simulink model "hydraulic_motor"  (R2013b)
settings: Solver=ode45  StartTime=0.0  StopTime=t_end  MaxStep=0.001  RelTol=1e-3
values from neighbouring files (symbols this model uses):
  b = 1e-3    (= 0.001)    [Hydraulic_script.m]
  C = 1e-12    [Hydraulic_script.m]
  I = 20000    [Hydraulic_script.m]
  J = r^2*100/(i^2)    (= 0.00907029478458)    [Hydraulic_script.m]
  P = 55000    [Hydraulic_script.m]
  target_angular_velocity = 210    [Hydraulic_script.m]
  Vr = 8.2e-6    (= 8.2e-06)    [Hydraulic_script.m]
settings Model: Creator=tlantela  LastModifiedBy=Tapio
settings OptimizationCC: SimCompilerOptimization=off
settings DebuggingCC: UnderspecifiedInitializationDetection=Simplified  MergeDetectMultiDrivingBlocksExec=error  FrameProcessingCompatibilityMsg=error
settings RTWCC: RTWCompilerOptimization=off
settings GRTTargetCC: TargetLangStandard=C89/C90 (ANSI)  CodeReplacementLibrary=None  CPPClassGenCompliant=on

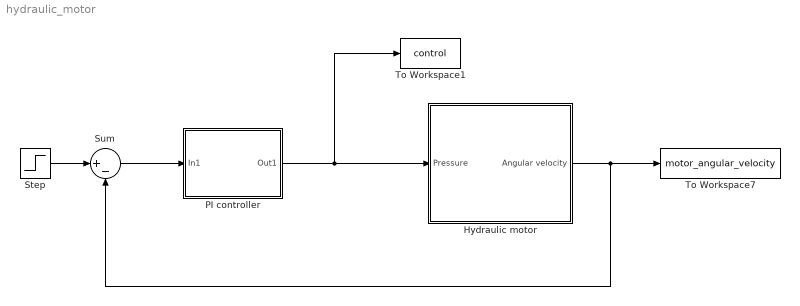
== system hydraulic_motor ==
  Hydraulic motor : Subsystem
  PI controller : Subsystem
  Step : Step  Time=0  After=target_angular_velocity  SampleTime=0
  Sum : Sum  Inputs=|+-
  To Workspace1 : ToWorkspace  VariableName=control  SampleTime=-1  SaveFormat=Timeseries
  To Workspace7 : ToWorkspace  VariableName=motor_angular_velocity  SampleTime=-1  SaveFormat=Timeseries
  wires:
  Hydraulic motor/1(Angular velocity) -> Sum/2, To Workspace7/1
  PI controller/1(Out1) -> Hydraulic motor/1(Pressure), To Workspace1/1
  Sum/1 -> PI controller/1(In1)
  Step/1 -> Sum/1

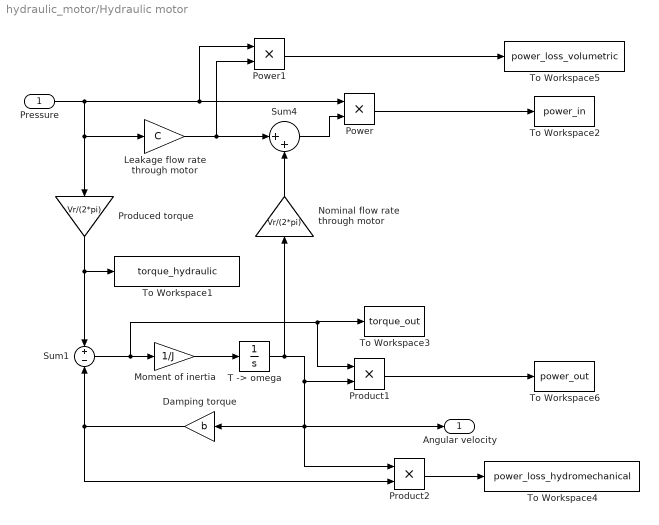
== system hydraulic_motor/Hydraulic motor ==
  Pressure : Inport
  Damping torque : Gain  Gain=b
  Leakage flow rate through motor : Gain  Gain=C
  Moment of inertia : Gain  Gain=1/J
  Nominal flow rate through motor : Gain  Gain=Vr/(2*pi)
  Power : Product
  Power1 : Product
  Produced torque : Gain  Gain=Vr/(2*pi)
  Product1 : Product
  Product2 : Product
  Sum1 : Sum  Inputs=+-
  Sum4 : Sum  Inputs=|++
  "T -> omega" : Integrator
  To Workspace1 : ToWorkspace  VariableName=torque_hydraulic  SampleTime=-1  SaveFormat=Timeseries
  To Workspace2 : ToWorkspace  VariableName=power_in  SampleTime=-1  SaveFormat=Timeseries
  To Workspace3 : ToWorkspace  VariableName=torque_out  SampleTime=-1  SaveFormat=Timeseries
  To Workspace4 : ToWorkspace  VariableName=power_loss_hydromechanical  SampleTime=-1  SaveFormat=Timeseries
  To Workspace5 : ToWorkspace  VariableName=power_loss_volumetric  SampleTime=-1  SaveFormat=Timeseries
  To Workspace6 : ToWorkspace  VariableName=power_out  SampleTime=-1  SaveFormat=Timeseries
  Angular velocity : Outport
  wires:
  Pressure/1 -> Leakage flow rate through motor/1, Produced torque/1, Power1/1, Power/1
  Moment of inertia/1 -> "T -> omega"/1
  Damping torque/1 -> Product2/2, Sum1/2
  Sum1/1 -> To Workspace3/1, Product1/1, Moment of inertia/1
  Product1/1 -> To Workspace6/1
  "T -> omega"/1 -> Product1/2, Damping torque/1, Product2/1, Angular velocity/1, Nominal flow rate through motor/1
  Power/1 -> To Workspace2/1
  Leakage flow rate through motor/1 -> Power1/2, Sum4/1
  Nominal flow rate through motor/1 -> Sum4/2
  Sum4/1 -> Power/2
  Power1/1 -> To Workspace5/1
  Product2/1 -> To Workspace4/1
  Produced torque/1 -> Sum1/1, To Workspace1/1

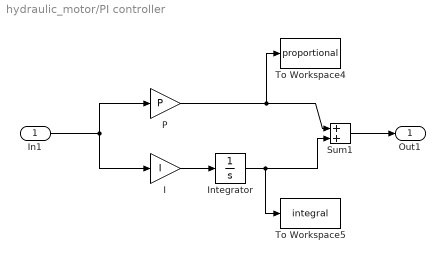
== system hydraulic_motor/PI controller ==
  In1 : Inport
  I : Gain  Gain=I
  Integrator : Integrator
  P : Gain  Gain=P
  Sum1 : Sum
  To Workspace4 : ToWorkspace  VariableName=proportional  SampleTime=-1  SaveFormat=Timeseries
  To Workspace5 : ToWorkspace  VariableName=integral  SampleTime=-1  SaveFormat=Timeseries
  Out1 : Outport
  wires:
  In1/1 -> I/1, P/1
  I/1 -> Integrator/1
  P/1 -> Sum1/1, To Workspace4/1
  Integrator/1 -> Sum1/2, To Workspace5/1
  Sum1/1 -> Out1/1
